simulink model "kinematic_bicycle"  (R2019a)
settings: Solver=VariableStepAuto  StartTime=0.0  StopTime=15  RelTol=1e-3
values from neighbouring files (symbols this model uses):
  init_states = [0; 0; 0; 0; 0;0;0]    [config_kinematic_bicycle.m]
  length_front = 0.8    [config_kinematic_bicycle.m]
  length_rear = 1.2    [config_kinematic_bicycle.m]
undefined symbols (not defined in the file or in its folder): velocity_angle
libraries: simulink_extras x1, simulink x1
settings Model: Creator=jacoboffersen  LastModifiedBy=jacoboffersen

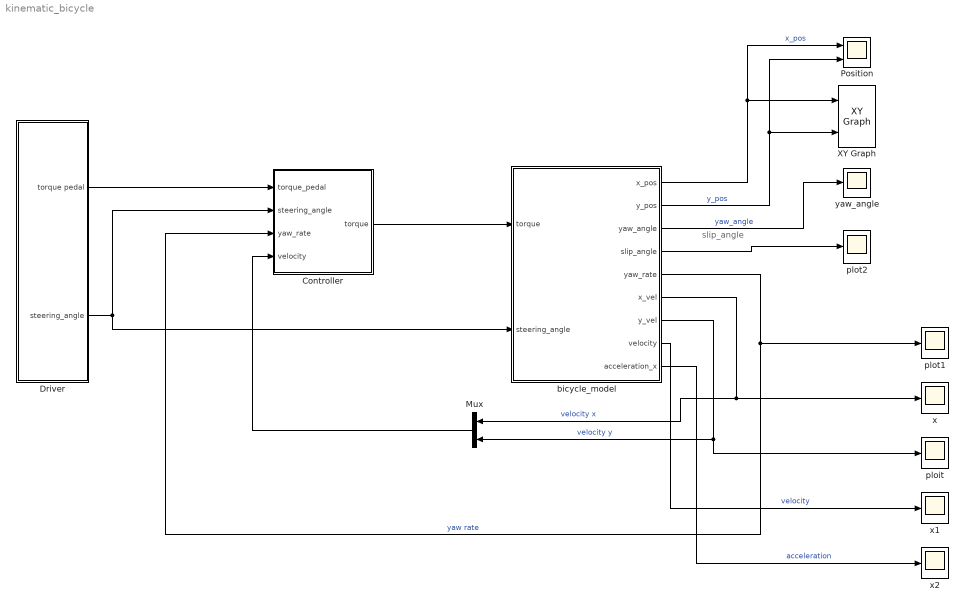
== system kinematic_bicycle ==
  note: slip_angle
  Controller : Subsystem
  Driver : Subsystem
  Mux : Mux  Inputs=2
  Position : Scope  NumInputPorts=2
  XY Graph : simulink/Sinks/XY Graph  xmin=-100  xmax=100  ymin=-100  ymax=100  st=0.01
  "bicycle_model " : Subsystem
  ploit : Scope
  plot1 : Scope
  plot2 : Scope
  x : Scope
  x1 : Scope
  x2 : Scope
  yaw_angle : Scope
  wires:
  "bicycle_model "/2(y_pos) -> XY Graph/2, Position/2  "y_pos"
  "bicycle_model "/1(x_pos) -> XY Graph/1, Position/1  "x_pos"
  "bicycle_model "/4(slip_angle) -> plot2/1
  "bicycle_model "/3(yaw_angle) -> yaw_angle/1  "yaw_angle"
  Driver/2(steering_angle) -> "bicycle_model "/2("steering_angle "), Controller/2(steering_angle)
  "bicycle_model "/5(yaw_rate) -> plot1/1, Controller/3(yaw_rate)  "yaw rate"
  "bicycle_model "/6(x_vel) -> Mux/1, x/1  "velocity x"
  "bicycle_model "/7(y_vel) -> Mux/2, ploit/1  "velocity y"
  Controller/1(torque) -> "bicycle_model "/1(torque)
  Driver/1(torque pedal) -> Controller/1(torque_pedal)
  Mux/1 -> Controller/4(velocity)
  "bicycle_model "/8(velocity) -> x1/1  "velocity"
  "bicycle_model "/9(acceleration_x) -> x2/1  "acceleration"

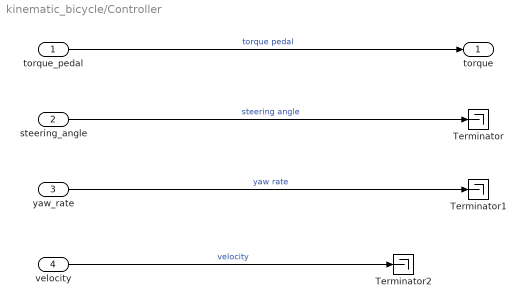
== system kinematic_bicycle/Controller ==
  torque_pedal : Inport
  steering_angle : Inport  Port=2
  yaw_rate : Inport  Port=3
  velocity : Inport  Port=4
  Terminator : Terminator
  Terminator1 : Terminator
  Terminator2 : Terminator
  torque : Outport
  wires:
  torque_pedal/1 -> torque/1  "torque pedal"
  steering_angle/1 -> Terminator/1  "steering angle"
  yaw_rate/1 -> Terminator1/1  "yaw rate"
  velocity/1 -> Terminator2/1  "velocity"

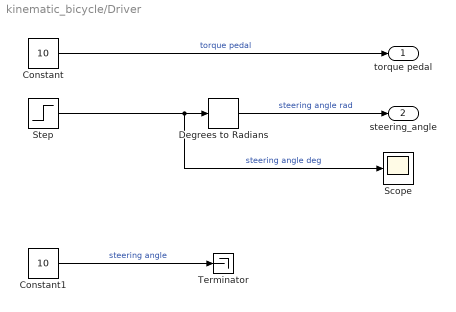
== system kinematic_bicycle/Driver ==
  Constant : Constant  Value=10
  Constant1 : Constant  Value=10
  Degrees to Radians : simulink_extras/Transformations/Degrees to Radians
  Scope : Scope
  Step : Step  Time=2  After=5  SampleTime=0
  Terminator : Terminator
  torque pedal : Outport
  steering_angle : Outport  Port=2
  wires:
  Constant/1 -> torque pedal/1  "torque pedal"
  Step/1 -> Scope/1, Degrees to Radians/1  "steering angle deg"
  Constant1/1 -> Terminator/1  "steering angle"
  Degrees to Radians/1 -> steering_angle/1  "steering angle rad"

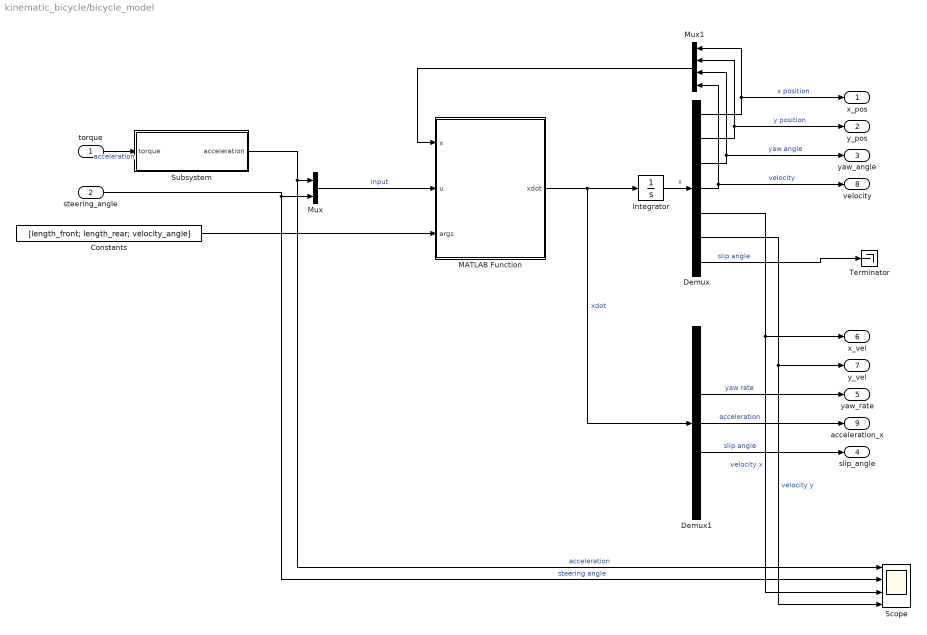
== system kinematic_bicycle/bicycle_model  ==
  torque : Inport
  "steering_angle " : Inport  Port=2
  Constants : Constant  Value=[length_front; length_rear; velocity_angle]
  Demux : Demux  Outputs=7
  Demux1 : Demux  Outputs=7
  Integrator : Integrator  InitialCondition=[init_states]
  MATLAB Function : MATLAB Function  TreatAsAtomicUnit=on
  Mux : Mux  Inputs=2
  Mux1 : Mux
  Scope : Scope  NumInputPorts=4
  Subsystem : Subsystem
  Terminator : Terminator
  x_pos : Outport
  y_pos : Outport  Port=2
  yaw_angle : Outport  Port=3
  slip_angle : Outport  Port=4
  yaw_rate : Outport  Port=5
  x_vel : Outport  Port=6
  y_vel : Outport  Port=7
  velocity : Outport  Port=8
  acceleration_x : Outport  Port=9
  wires:
  Mux/1 -> MATLAB Function/2(u)  "input"
  "steering_angle "/1 -> Scope/2, Mux/2  "steering angle"
  Constants/1 -> MATLAB Function/3(args)
  MATLAB Function/1(xdot) -> Demux1/1, Integrator/1  "xdot"
  Integrator/1 -> Demux/1  "x"
  Demux/1 -> x_pos/1, Mux1/1  "x position"
  Demux/2 -> y_pos/1, Mux1/2  "y position"
  Demux/3 -> yaw_angle/1, Mux1/3  "yaw angle"
  Demux1/5 -> slip_angle/1  "slip angle"
  Mux1/1 -> MATLAB Function/1(x)
  Demux1/3 -> yaw_rate/1  "yaw rate"
  Demux/5 -> Scope/3, x_vel/1  "velocity x"
  Demux1/4 -> acceleration_x/1  "acceleration"
  Demux/4 -> velocity/1, Mux1/4  "velocity"
  Demux/6 -> Scope/4, y_vel/1  "velocity y"
  Demux/7 -> Terminator/1  "slip angle"
  Subsystem/1(acceleration) -> Scope/1, Mux/1  "acceleration"
  torque/1 -> Subsystem/1(torque)  "acceleration"

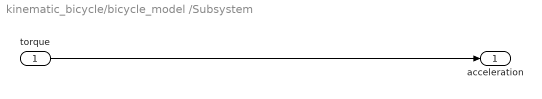
== system kinematic_bicycle/bicycle_model /Subsystem ==
  torque : Inport
  acceleration : Outport
  wires:
  torque/1 -> acceleration/1

== matlab function kinematic_bicycle/bicycle_model /MATLAB Function ==
  data: x input; xdot output; u input; args input
function xdot = fcn(x, u, args)

x_pos            = x(1); % x pos
y_pos            = x(2); % y pos
yaw_angle        = x(3); % Yaw angle
velocity         = x(4); % Velocity

acceleration         = u(1); % Velocity
steering_angle   = u(2); % Steering angle

length_front     = args(1); % Length from front axle to CG
length_rear      = args(2); % Length fromt rear axle to CG
% velocity_angle   = args(3); % Angle of velocity

slip_angle = atan(length_rear * tan(steering_angle) / (length_front + length_rear));

x_change = velocity * cos(yaw_angle + slip_angle);
y_change = velocity * sin(yaw_angle + slip_angle);
velocity_x = velocity * cos(slip_angle);
velocity_y = velocity * sin(slip_angle);
yaw_rate = tan(steering_angle) * (velocity * cos(slip_angle))/(length_front + length_rear);

xdot = [x_change; y_change; yaw_rate; acceleration;velocity_x; velocity_y; slip_angle];
